simulink model "routeTracking"  (R2014b)
settings: Solver=ode45  StartTime=0.0  StopTime=10.0  RelTol=1e-3
settings Model: Creator=Think  LastModifiedBy=Think

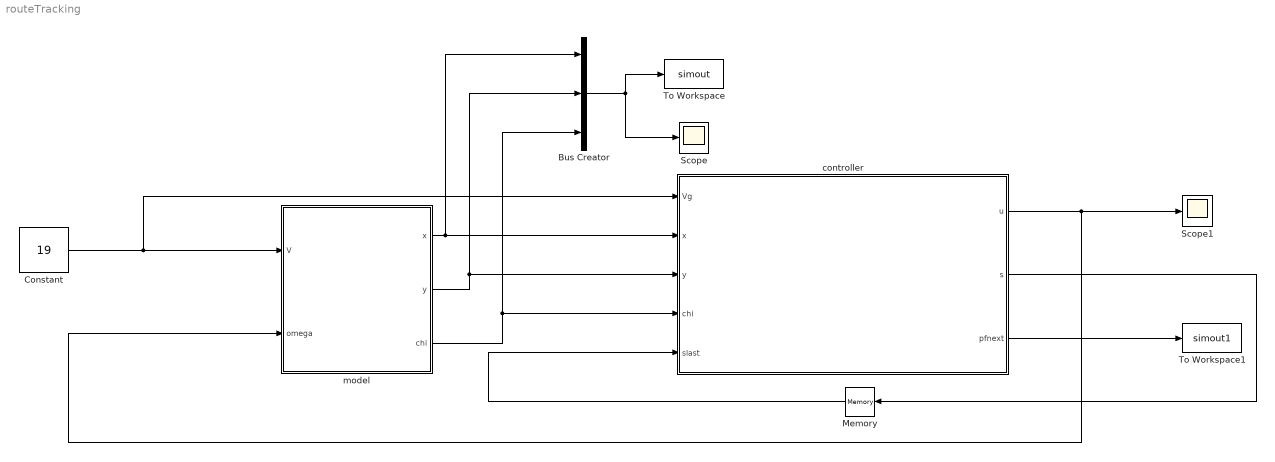
== system routeTracking ==
  Bus Creator : BusCreator  Inputs=3
  Constant : Constant  Value=19
  Memory : Memory
  Scope : Scope
      settings: YMin=-150  YMax=250
  Scope1 : Scope
      settings: YMin=-1250  YMax=1250
  To Workspace : ToWorkspace  VariableName=simout  SaveFormat=Timeseries  SampleTime=-1
  To Workspace1 : ToWorkspace  VariableName=simout1  SaveFormat=Timeseries  SampleTime=-1
  controller : MATLAB Function  TreatAsAtomicUnit=on
  model : Subsystem
  wires:
  Bus Creator/1 -> Scope/1, To Workspace/1
  controller/2(s) -> Memory/1
  Memory/1 -> controller/5(slast)
  controller/3(pfnext) -> To Workspace1/1
  model/1(x) -> Bus Creator/1, controller/2(x)
  model/2(y) -> Bus Creator/2, controller/3(y)
  model/3(chi) -> Bus Creator/3, controller/4(chi)
  controller/1(u) -> Scope1/1, model/2(omega)
  Constant/1 -> controller/1(Vg), model/1(V)

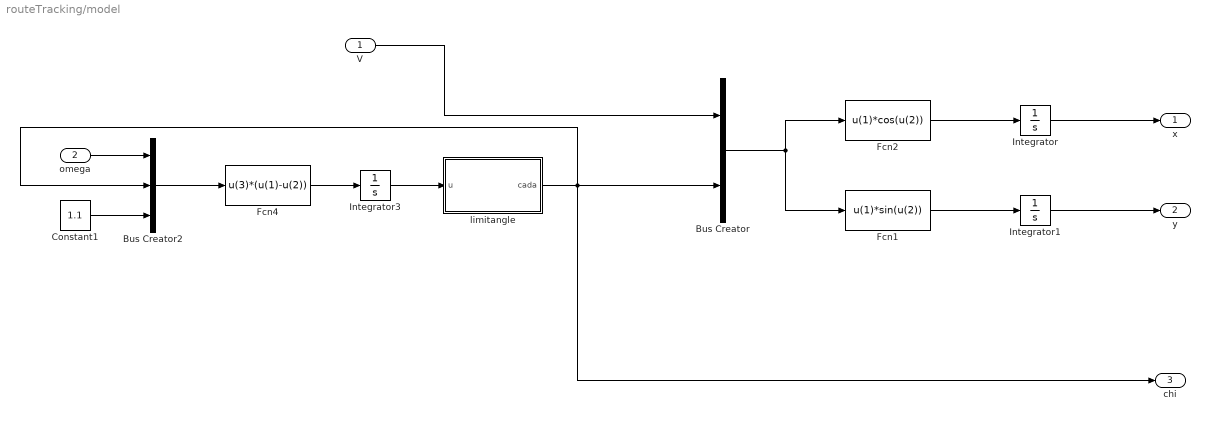
== system routeTracking/model ==
  V : Inport
  omega : Inport  Port=2
  Bus Creator : BusCreator  Inputs=2
  Bus Creator2 : BusCreator  Inputs=3
  Constant1 : Constant  Value=1.1
  Fcn1 : Fcn  Expr=u(1)*sin(u(2))
  Fcn2 : Fcn  Expr=u(1)*cos(u(2))
  Fcn4 : Fcn  Expr=u(3)*(u(1)-u(2))
  Integrator : Integrator
  Integrator1 : Integrator  InitialCondition=10
  Integrator3 : Integrator
  limitangle : MATLAB Function  TreatAsAtomicUnit=on
  x : Outport
  y : Outport  Port=2
  chi : Outport  Port=3
  wires:
  Integrator/1 -> x/1
  Integrator1/1 -> y/1
  V/1 -> Bus Creator/1
  Fcn2/1 -> Integrator/1
  Integrator3/1 -> limitangle/1(u)
  Bus Creator/1 -> Fcn1/1, Fcn2/1
  Fcn1/1 -> Integrator1/1
  omega/1 -> Bus Creator2/1
  Constant1/1 -> Bus Creator2/3
  Bus Creator2/1 -> Fcn4/1
  Fcn4/1 -> Integrator3/1
  limitangle/1(cada) -> Bus Creator2/2, Bus Creator/2, chi/1

== matlab function routeTracking/controller ==
  data: Vg input; x input; y input; u output; chi input; slast input; s output; pfnext output
function [u,s,pfnext]= fcn(Vg,x,y,chi,slast)
% %% parameters setting

%#eml
%% setting ,
p=[x,y];
L=30;
%% control law
[pfnext,chif,s,ydis]=getnearestposition(L,p,slast);

%k=0.2;
kappa=10;
epsilon=1;

% tchi=chi-chif;
% if tchi>pi
%     tchi=tchi-2*pi;
% elseif tchi<-pi
%     tchi=tchi+2*pi;
% end
%     
error=[cos(chif) -sin(chif);sin(chif) cos(chif)]'*(p'-pfnext');
es=error(1);
ed=error(2);

ydis=error(2);

%ydis=2*(-x+y)/sqrt(2);
%ydis=y;
%chidy=-chiinf*(2/pi)*atan(k*ydis);
%%
chiinf=pi/4;
k=0.01;
chidy=-chiinf*(exp(2*k*ed)-1)/(exp(2*k*ed)+1); %%approach angle
tchi=chi-chidy;
if tchi>pi
    tchi=tchi-2*pi;
elseif tchi<-pi
    tchi=tchi+2*pi;
end
u=chi-(1/1.1)*chiinf*(2/pi)*(k/(1+k*k*ydis*ydis))*Vg*sin(chi)-1/1.1*kappa*sat(tchi/epsilon);

while u>pi
   u = u-2*pi;
end

while u<-pi
   u = u+2*pi;
end



function [pf,chif]=curvefun(s)  %曲线参数方程
%     %% 此处以圆为例
   R=200;
   Ocenter=[-200,0];
   theta=s/R;
   pfx=R*cos(theta)+Ocenter(1);
   pfy=R*sin(theta)+Ocenter(2);
   pf=[pfx,pfy];
   
   xprim=-sin(theta);
   yprim=cos(theta);
   
   %% 此处以直线为例
%    initp=[0,0];
%    alpha=pi/3;
%    pfx=s*cos(alpha)+initp(1);
%    pfy=s*sin(alpha)+initp(2);
%       
%    pf=[pfx,pfy];
% %     % 
%    xprim=cos(alpha);
%    yprim=sin(alpha);

% % 
  chif=atan(yprim/xprim);



 function [pf,chif,mins,mindis]=getnearestposition(L,p,sinput)
     ssample=0.1;
     N=2*L/ssample;
     mindis=norm(p-curvefun(sinput));
     mins=sinput;
     [pf,chif]=curvefun(sinput);
     
     for i=0:N
         site=sinput-L+i*ssample;
         [pite,chifite]=curvefun(site);
         dis=norm(p-pite);
         if(dis<mindis)
             mindis=dis;
             mins=site;
             pf=pite;
             chif=chifite;
         end
     end
     
     function y=sat(x)
         if abs(x)<=1
             y=x;
         else
             y=sign(x);
         end

== matlab function routeTracking/model/limitangle ==
  data: u input; cada output
function cada  = limitminpi2pi(u)
%#codegen

while u>pi
   u = u-2*pi;
end

while u<-pi
   u = u+2*pi;
end

    cada=u;
